simulink model "OnestepMovement"  (R2018b)
settings: Solver=FixedStepDiscrete  StartTime=0.0  StopTime=inf  RelTol=1e-3
undefined symbols (not defined in the file): Angular, Linear
libraries: robotlib x4
settings Model: Creator=Kim Hyup  LastModifiedBy=Kim Hyup

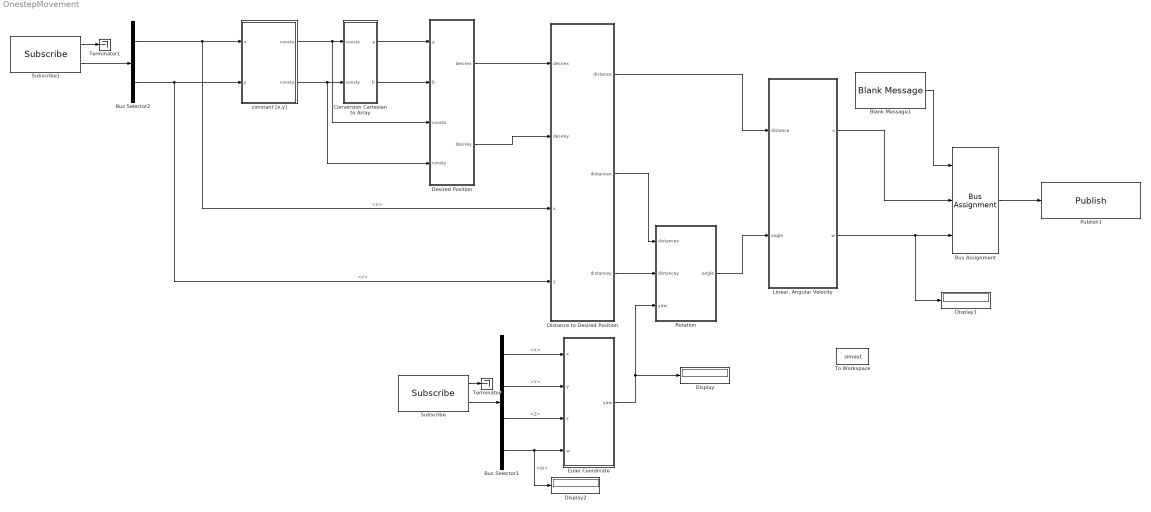
== system OnestepMovement ==
  Blank Message1 : robotlib/Blank Message  messageClass=Message  entityType=geometry_msgs/Twist  messageType=geometry_msgs/Twist  SampleTime=inf
      settings: SourceProductBaseCode=RO
  Bus Assignment : BusAssignment  AssignedSignals=Linear.X,Angular.Z
  Bus Selector1 : BusSelector  OutputSignals=Pose.Pose.Orientation.X,Pose.Pose.Orientation.Y,Pose.Pose.Orientation.Z,Pose.Pose.Orientation.W
  Bus Selector2 : BusSelector  OutputSignals=Pose.Pose.Position.X,Pose.Pose.Position.Y
  Conversion Cartesian to Array : MATLAB Function  TreatAsAtomicUnit=on
  Desired Position : MATLAB Function  TreatAsAtomicUnit=on
  Display : Display
  Display1 : Display
  Display2 : Display
  Distance to Desired Position : MATLAB Function  TreatAsAtomicUnit=on
  Euler Coordinate : MATLAB Function  TreatAsAtomicUnit=on
  "Linear, Angular Velocity" : MATLAB Function  TreatAsAtomicUnit=on
  Publish1 : robotlib/Publish  topicSource=Select from ROS network  topic=/mobile_base/commands/velocity  messageType=geometry_msgs/Twist  messageQueueLength=1
      settings: SourceProductBaseCode=RO
  Rotation : MATLAB Function  TreatAsAtomicUnit=on
  Subscribe : robotlib/Subscribe  topicSource=Select from ROS network  topic=/odom  messageType=nav_msgs/Odometry  sampleTime=-1  messageQueueLength=1
      settings: SourceProductBaseCode=RO
  Subscribe1 : robotlib/Subscribe  topicSource=Select from ROS network  topic=/odom  messageType=nav_msgs/Odometry  sampleTime=-1  messageQueueLength=1
      settings: SourceProductBaseCode=RO
  Terminator : Terminator
  Terminator1 : Terminator
  To Workspace : ToWorkspace  VariableName=simout  SaveFormat=Timeseries  SampleTime=-1
  constant [x,y] : MATLAB Function  TreatAsAtomicUnit=on
  wires:
  Subscribe/2 -> Bus Selector1/1
  Bus Selector1/1 -> Euler Coordinate/1(x)  "<X>"
  Bus Selector1/2 -> Euler Coordinate/2(y)  "<Y>"
  Bus Selector1/3 -> Euler Coordinate/3(z)  "<Z>"
  Bus Selector1/4 -> Display2/1, Euler Coordinate/4(w)  "<W>"
  Blank Message1/1 -> Bus Assignment/1
  Bus Assignment/1 -> Publish1/1
  Subscribe1/2 -> Bus Selector2/1
  Bus Selector2/1 -> Distance to Desired Position/3(x), constant [x,y]/1(x)  "<X>"
  Bus Selector2/2 -> Distance to Desired Position/4(y), constant [x,y]/2(y)  "<Y>"
  constant [x,y]/2(consty) -> Desired Position/4(consty), Conversion Cartesian to Array/2(consty)
  constant [x,y]/1(constx) -> Desired Position/3(constx), Conversion Cartesian to Array/1(constx)
  Conversion Cartesian to Array/1(a) -> Desired Position/1(a)
  Conversion Cartesian to Array/2(b) -> Desired Position/2(b)
  Desired Position/1(desirex) -> Distance to Desired Position/1(desirex)
  Desired Position/2(desirey) -> Distance to Desired Position/2(desirey)
  Euler Coordinate/1(yaw) -> Display/1, Rotation/3(yaw)
  Distance to Desired Position/2(distancex) -> Rotation/1(distancex)
  Distance to Desired Position/3(distancey) -> Rotation/2(distancey)
  Distance to Desired Position/1(distance) -> "Linear, Angular Velocity"/1(distance)
  Rotation/1(angle) -> "Linear, Angular Velocity"/2(angle)
  "Linear, Angular Velocity"/1(v) -> Bus Assignment/2
  "Linear, Angular Velocity"/2(w) -> Display1/1, Bus Assignment/3
  Subscribe/1 -> Terminator/1
  Subscribe1/1 -> Terminator1/1

== matlab function OnestepMovement/constant [x,y] ==
  data: x input; constx output; y input; consty output
function [constx,consty] = constant(x,y)

if (x >= 0) && (x < 3)
    constx = 1;
elseif (x >= 3) && (x < 5)
    constx = 3;
elseif (x >= 5) && (x < 7)
    constx = 5;
else
    constx = 7;
end

if (y >= 0) && (y < 3)
    consty = 1;
elseif (y >= 3) && (y < 5)
    consty = 3;
elseif (y >= 5) && (y < 7)
    consty = 5;
else
    consty = 7;
end

== matlab function OnestepMovement/Euler Coordinate ==
  data: x input; yaw output; y input; z input; w input
function yaw = quat2eul(x,y,z,w)

eul = quat2eul([w,x,y,z]);
yaw = eul(1);

end

== matlab function OnestepMovement/Desired Position ==
  data: a input; desirex output; b input; constx input; consty input; desirey output
function [desirex,desirey] = movement(a,b,constx,consty)
num_states = [1 2 3 4 3 2 1];
costs = zeros([7 7 7 7]);
costs(1,1,2,1) = 1;
costs(1,1,2,2) = 10;
costs(2,1,3,1) = 10;
costs(2,1,3,2) = 1;
costs(2,2,3,2) = 1;
costs(2,2,3,3) = 1;
costs(3,1,4,1) = 10;
costs(3,1,4,2) = 1;
costs(3,2,4,2) = 1;
costs(3,2,4,3) = 10;
costs(3,3,4,3) = 1;
costs(3,3,4,4) = 10;
costs(4,1,5,1) = 1;
costs(4,2,5,1) = 1;
costs(4,2,5,2) = 1;
costs(4,3,5,2) = 10;
costs(4,3,5,3) = 1;
costs(4,4,5,3) = 1;
costs(5,1,6,1) = 10;
costs(5,2,6,1) = 1;
costs(5,2,6,2) = 1;
costs(5,3,6,2) = 1;
costs(6,1,7,1) = 1;
costs(6,2,7,1) = 10;

costs(2,1,3,3) = 20;
costs(2,2,3,1) = 20;
costs(3,1,4,3) = 20;
costs(3,1,4,4) = 20;
costs(3,2,4,1) = 20;
costs(3,2,4,4) = 20;
costs(3,3,4,1) = 20;
costs(3,3,4,2) = 20;
costs(4,1,5,2) = 20;
costs(4,1,5,3) = 20;
costs(4,2,5,3) = 20;
costs(4,3,5,1) = 20;
costs(4,4,5,1) = 20;
costs(4,4,5,2) = 20;
costs(5,1,6,2) = 20;
costs(5,3,6,1) = 20;

V = zeros([7 4]);
d = costs;
V(7,1)=0;
for k=6:-1:1
 for i=1:num_states(k)
    path_length = zeros([1 num_states(k+1)]);
    for j=1:num_states(k+1)
        path_length(j)= d(k,i,k+1,j)+V(k+1,j);
    end
 V(k,i)=min(path_length);
 end
end

path_way = zeros([1 2]);
if a == 7
    desirex = 7;
    desirey = 7;
elseif b == 4
    desirex = constx;
    desirey = consty + 2;
else
    path_way(1) = d(a,b,a+1,b) + V(a+1,b);
    path_way(2) = d(a,b,a+1,b+1) + V(a+1,b+1);
    [~,index] = min(path_way);
    if index == 1
        desirex = constx;
        desirey = consty + 2;
    else
        desirex = constx +2;
        desirey = consty;
    end
end

== matlab function OnestepMovement/Conversion Cartesian to Array ==
  data: constx input; a output; consty input; b output
function [a,b] = carte2array(constx,consty)

if (constx == 1) && (consty == 1)
    a = 1;
    b = 1;
elseif (constx == 1) && (consty == 3)
    a = 2;
    b = 1;
elseif (constx == 3) && (consty == 1)
    a = 2;
    b = 2;
elseif (constx == 1) && (consty == 5)
    a = 3;
    b = 1;
elseif (constx == 3) && (consty == 3)
    a = 3;
    b = 2;
elseif (constx == 5) && (consty == 1)
    a = 3;
    b = 3;
elseif (constx == 1) && (consty == 7)
    a = 4;
    b = 1;
elseif (constx == 3) && (consty == 5)
    a = 4;
    b = 2;
elseif (constx == 5) && (consty == 3)
    a = 4;
    b = 3;
elseif (constx == 7) && (consty == 1)
    a = 4;
    b = 4;
elseif (constx == 3) && (consty == 7)
    a = 5;
    b = 1;
elseif (constx == 5) && (consty == 5)
    a = 5;
    b = 2;
elseif (constx == 7) && (consty == 3)
    a = 5;
    b = 3;
elseif (constx == 5) && (consty == 7)
    a = 6;
    b = 1;
elseif (constx == 7) && (consty == 5)
    a = 6;
    b = 2;
else
    a = 7;
    b = 1;
end

== matlab function OnestepMovement/Rotation ==
  data: distancex input; angle output; distancey input; yaw input
function angle = angle(distancex,distancey,yaw)

desireangle = atan2(distancey,distancex);
u = desireangle - yaw;
angle = abs(u);

== matlab function OnestepMovement/Distance to Desired Position ==
  data: distance output; desirex input; distancex output; desirey input; x input; y input; distancey output
function [distance,distancex,distancey] = distance(desirex,desirey,x,y)

distancex = desirex - x;
distancey = desirey - y;
distance = sqrt(distancex^2 + distancey^2);

== matlab function OnestepMovement/Linear, Angular Velocity ==
  data: distance input; v output; angle input; w output
function [v,w] = velocity(distance,angle)

if (angle <= 0.5) %% w = angular velocity
    w = 0;
else
    w = 0.5;
end

if (w == 0)
    if (distance <= 0.5) %% v = linear velocity
        v = 0;
    else
        v = 1;
    end
else
    v = 0;
end
